simulink model "fir_model"  (R2021a)
settings: Solver=FixedStepDiscrete  StartTime=0.0  StopTime=100  FixedStep=1  RelTol=1e-3
settings Model: Creator=user  LastModifiedBy=user

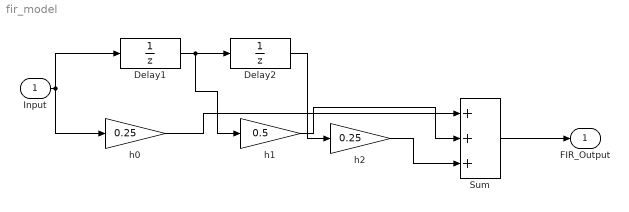
== system fir_model ==
  Input : Inport
  Delay1 : UnitDelay  HasFrameUpgradeWarning=on
  Delay2 : UnitDelay  HasFrameUpgradeWarning=on
  Sum : Sum  Inputs=+++
  h0 : Gain  Gain=0.25
  h1 : Gain  Gain=0.5
  h2 : Gain  Gain=0.25
  FIR_Output : Outport
  wires:
  Input/1 -> Delay1/1, h0/1
  Delay1/1 -> Delay2/1, h1/1
  Delay2/1 -> h2/1
  h0/1 -> Sum/1
  h1/1 -> Sum/2
  h2/1 -> Sum/3
  Sum/1 -> FIR_Output/1
